simulink model "Batteryfault"  (R2021a)
settings: Solver=ode23t  StartTime=0.0  StopTime=50  RelTol=1e-3
libraries: ee_lib x40, fl_lib x12, nesl_utility x3
settings Model: Creator=perry  LastModifiedBy=perry

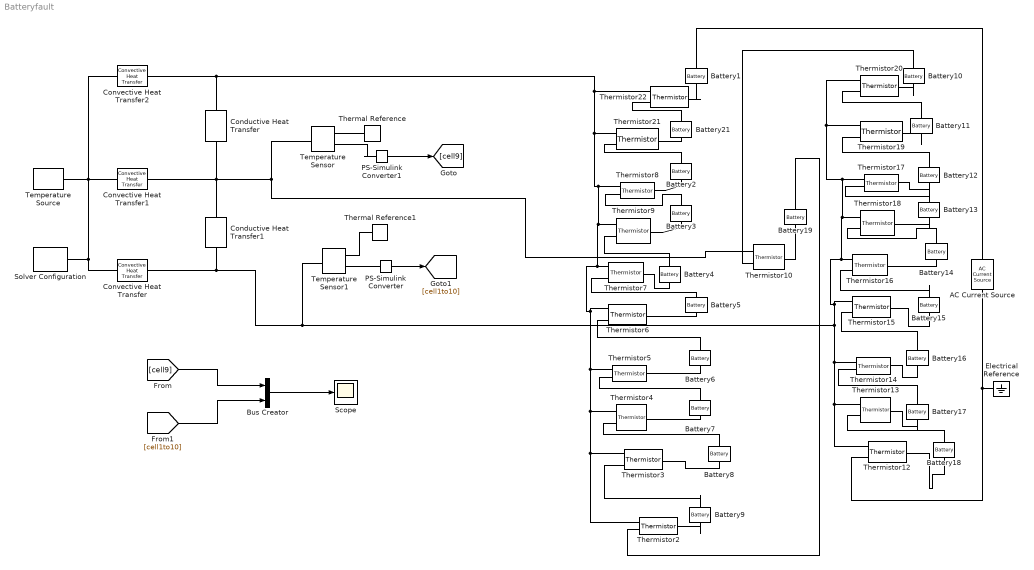
== system Batteryfault ==
  AC Current Source : fl_lib/Electrical/Electrical Sources/AC Current Source  amp=50 A  shift=0 deg  frequency=1/600 Hz  omega=0 rad/s
      settings: SourceProductBaseCode=SS  InternalSimscapePortConfiguration="{\"Bottom\":[],\"Left\":[{\"id\":\"p\",\"label\":\"\",\"type\":\"foundation.electrical.electrical\"}],\"Right\":[{\"id\":\"n\",\"label\":\"\",\"type\":\"foundation.electrical.electrical\"}],\"Top\":[]}"
  Battery{1..19,21} (20 alike) : ee_lib/Sources/Battery  Vnom=4 V  prm_dir=1  R1_dis=2 Ohm  R1_ch=2 Ohm  R1=0.001 Ohm  prm_AH=2  AH=5 hr*A  V1=3.6 V  AH1=4 hr*A  prm_R2=1  R2=2000 Ohm  prm_dyn=1  Rp1=0.005 Ohm  tau1=30 s  Rp2=0.005 Ohm  tau2=30 s  Rp3=0.005 Ohm  tau3=30 s  Rp4=0.005 Ohm  tau4=30 s  Rp5=0.005 Ohm  tau5=30 s  prm_fade=1  N_fade=100  AH_fade=45 hr*A  R1_fade=2.02 Ohm  R1_ch_fade=2.02 Ohm  V1_fade=10.35 V  prm_age=1  prm_age_OCV=1  OCV_age=0.9  SOC_age=60  Tmeas_age=298.15 K  delta_time_age_vec=[0] d  temperature_age_vec=[273] K  OCV_scaling_age=2.2134e6  OCV_offset_age=1.632e6  temp_exp_age=0.515833569 V  t_exp_age=0.75  i_specify=off  i_priority=None  i=0 A  i_nominal_specify=off  i_nominal_unit=A  i_nominal_value=1  v_specify=off  v_priority=None  v=0 V  v_nominal_specify=off  v_nominal_unit=V  v_nominal_value=1  charge_specify=off  charge_priority=High  charge=50 hr*A  charge_nominal_specify=off  charge_nominal_unit=hr*A  charge_nominal_value=1  num_cycles_specify=off  num_cycles_priority=High  num_cycles=0  num_cycles_nominal_specify=off  num_cycles_nominal_unit=1  num_cycles_nominal_value=1  thermal_mass=30000 J/K  Tmeas=298.15 K  Vnom_T2=12 V  R1_T2=2.2 Ohm  R1_T2_dis=2.2 Ohm  R1_T2_ch=2.2 Ohm  V1_T2=11.4 V  R2_T2=2200 Ohm  Rp1_T2=0.005 Ohm  tau1_T2=30 s  Rp2_T2=0.005 Ohm  tau2_T2=30 s  Rp3_T2=0.005 Ohm  tau3_T2=30 s  Rp4_T2=0.005 Ohm  tau4_T2=30 s  Rp5_T2=0.005 Ohm  tau5_T2=30 s  Tmeas2=273.15 K  temperature_specify=off  temperature_priority=High  temperature=298.15 K  temperature_nominal_specify=off  temperature_nominal_unit=K  temperature_nominal_value=1
      settings: SourceProductBaseCode=SN
  Bus Creator : BusCreator  Inputs=2
  Conductive Heat Transfer : fl_lib/Thermal/Thermal Elements/Conductive Heat Transfer  area=1e-4 m^2  thickness=0.1 m  th_cond=401 W/(m*K)  T_specify=off  T_priority=None  T=0 K  T_nominal_specify=off  T_nominal_unit=K  T_nominal_value=1  Q_specify=off  Q_priority=None  Q=0 W  Q_nominal_specify=off  Q_nominal_unit=W  Q_nominal_value=1
  Conductive Heat Transfer1 : fl_lib/Thermal/Thermal Elements/Conductive Heat Transfer  area=1e-4 m^2  thickness=0.1 m  th_cond=401 W/(m*K)  T_specify=off  T_priority=None  T=0 K  T_nominal_specify=off  T_nominal_unit=K  T_nominal_value=1  Q_specify=off  Q_priority=None  Q=0 W  Q_nominal_specify=off  Q_nominal_unit=W  Q_nominal_value=1
  Convective Heat Transfer : fl_lib/Thermal/Thermal Elements/Convective Heat Transfer  area=1e-4 m^2  heat_tr_coeff=20 W/(m^2 * K)  T_specify=off  T_priority=None  T=0 K  T_nominal_specify=off  T_nominal_unit=K  T_nominal_value=1  Q_specify=off  Q_priority=None  Q=0 W  Q_nominal_specify=off  Q_nominal_unit=W  Q_nominal_value=1
  Convective Heat Transfer1 : fl_lib/Thermal/Thermal Elements/Convective Heat Transfer  area=1e-4 m^2  heat_tr_coeff=20 W/(m^2 * K)  T_specify=off  T_priority=None  T=0 K  T_nominal_specify=off  T_nominal_unit=K  T_nominal_value=1  Q_specify=off  Q_priority=None  Q=0 W  Q_nominal_specify=off  Q_nominal_unit=W  Q_nominal_value=1
  Convective Heat Transfer2 : fl_lib/Thermal/Thermal Elements/Convective Heat Transfer  area=1e-4 m^2  heat_tr_coeff=20 W/(m^2 * K)  T_specify=off  T_priority=None  T=0 K  T_nominal_specify=off  T_nominal_unit=K  T_nominal_value=1  Q_specify=off  Q_priority=None  Q=0 W  Q_nominal_specify=off  Q_nominal_unit=W  Q_nominal_value=1
  Electrical Reference : fl_lib/Electrical/Electrical Elements/Electrical Reference
  PS-Simulink Converter : nesl_utility/PS-Simulink Converter  PhysicalDomain=network_engine_domain  SubClassName=ps_output  LeftPortType=input  RightPortType=output  PseudoPeriodic=off  Frequencies=[]  Unit=inherit  AffineConversion=off
      settings: SourceProductBaseCode=PW,SS
  PS-Simulink Converter1 : nesl_utility/PS-Simulink Converter  PhysicalDomain=network_engine_domain  SubClassName=ps_output  LeftPortType=input  RightPortType=output  PseudoPeriodic=off  Frequencies=[]  Unit=inherit  AffineConversion=off
      settings: SourceProductBaseCode=PW,SS
  Scope : Scope
  Solver Configuration : nesl_utility/Solver Configuration  PhysicalDomain=network_engine_domain  SubClassName=solver  LeftPortType=input  RightPortType=generic  Tones=[]  Harmonics=[]  SimulateNoise=off  Profile=off  UseLocalSampling=off  EnableSwitchedLinearOptims=on  FrequencyDomain=off  UseCCode=off  RelTol=0.001  AbsTol=1e-06  MinStep=1e-09  ToWorkspace=off  RevertToSquareIcSolve=off  NumHomotopyIterations=100  PhasorMode=off  PhasorModeNumHarmonics=1  DoDC=off  ResidualTolerance=1e-09  UseLocalSolver=off  LocalSolverChoice=NE_BACKWARD_EULER_ADVANCER  LocalSolverSampleTime=0.001  DoFixedCost=off  MaxNonlinIter=3  MaxModeIter=2  ComputeImpulses=off  ImpulseIterations=2  LinearAlgebra=Sparse  EquationFormulation=NE_TIME_EF  DelaysMemoryBudget=1024  AutomaticFiltering=on  FilteringTimeConstant=0.001  PartitionStorageMethod=AS_NEEDED  PartitionMemoryBudget=1024  PartitionMethod=ROBUST
      settings: SourceProductBaseCode=PW,SS
  Temperature Sensor : fl_lib/Thermal/Thermal Sensors/Temperature Sensor
  Temperature Sensor1 : fl_lib/Thermal/Thermal Sensors/Temperature Sensor
  Temperature Source : fl_lib/Thermal/Thermal Sources/Temperature Source  temperature=298 K
  Thermal Reference : fl_lib/Thermal/Thermal Elements/Thermal Reference
  Thermal Reference1 : fl_lib/Thermal/Thermal Elements/Thermal Reference
  Thermistor10 : ee_lib/Sensors & Transducers/Thermistor  R0=1000 Ohm  Bparam=3000 degC  T0=23 degC  tc=5.0 s  K_d=0.75e-3 W/K  T_specify=off  T_priority=High  T=298.15 K  T_nominal_specify=off  T_nominal_unit=K  T_nominal_value=1
      settings: SourceProductBaseCode=PS  InternalSimscapePortConfiguration="{\"Bottom\":[],\"Left\":[{\"id\":\"A\",\"label\":\"A\",\"type\":\"foundation.thermal.thermal\"},{\"id\":\"p\",\"label\":\"+\",\"type\":\"foundation.electrical.electrical\"}],\"Right\":[{\"id\":\"n\",\"label\":\"-\",\"type\":\"foundation.electrical.electrical\"}],\"Top\":[]}"
  Thermistor{2..9,12..22} (19 alike) : ee_lib/Sensors & Transducers/Thermistor  R0=1000 Ohm  Bparam=3000 degC  T0=25 degC  tc=5.0 s  K_d=0.75e-3 W/K  T_specify=off  T_priority=High  T=298.15 K  T_nominal_specify=off  T_nominal_unit=K  T_nominal_value=1
      settings: SourceProductBaseCode=PS  InternalSimscapePortConfiguration="{\"Bottom\":[],\"Left\":[{\"id\":\"A\",\"label\":\"A\",\"type\":\"foundation.thermal.thermal\"},{\"id\":\"p\",\"label\":\"+\",\"type\":\"foundation.electrical.electrical\"}],\"Right\":[{\"id\":\"n\",\"label\":\"-\",\"type\":\"foundation.electrical.electrical\"}],\"Top\":[]}"
  wires:
  PS-Simulink Converter1/1 -> [cell9]
  PS-Simulink Converter/1 -> [cell1to10]
  Bus Creator/1 -> Scope/1
  [cell9] -> Bus Creator/1
  [cell1to10] -> Bus Creator/2
  connections:
  Temperature Sensor1/RConn1 -- Thermal Reference1/LConn1
  Temperature Sensor1/RConn2 -- PS-Simulink Converter/LConn1
  Temperature Sensor/RConn1 -- Thermal Reference/LConn1
  PS-Simulink Converter1/LConn1 -- Temperature Sensor/RConn2
  Solver Configuration/RConn1 -- Convective Heat Transfer2/LConn1 -- Convective Heat Transfer1/LConn1 -- Temperature Source/LConn1 -- Convective Heat Transfer/LConn1
  Battery10/LConn1 -- Thermistor10/LConn2
  Battery10/RConn1 -- Thermistor20/RConn1
  Battery11/LConn1 -- Thermistor20/LConn2
  Battery11/RConn1 -- Thermistor19/RConn1
  Battery12/LConn1 -- Thermistor19/LConn2
  Thermistor17/RConn1 -- Battery12/RConn1
  Battery13/LConn1 -- Thermistor17/LConn2
  Battery13/RConn1 -- Thermistor18/RConn1
  Battery15/LConn1 -- Thermistor16/LConn2
  Battery15/RConn1 -- Thermistor15/RConn1
  Battery16/LConn1 -- Thermistor15/LConn2
  Battery16/RConn1 -- Thermistor14/RConn1
  Battery17/LConn1 -- Thermistor14/LConn2
  Battery17/RConn1 -- Thermistor13/RConn1
  Battery18/LConn1 -- Thermistor13/LConn2
  Battery18/RConn1 -- Thermistor12/RConn1
  AC Current Source/RConn1 -- Thermistor12/LConn2 -- Electrical Reference/LConn1
  Thermistor20/LConn1 -- Thermistor19/LConn1 -- Thermistor17/LConn1 -- Temperature Sensor1/LConn1 -- Convective Heat Transfer/RConn1 -- Conductive Heat Transfer1/RConn1 -- Thermistor12/LConn1 -- Thermistor13/LConn1 -- Thermistor14/LConn1 -- Thermistor15/LConn1 -- Thermistor16/LConn1 -- Thermistor18/LConn1
  Thermistor7/LConn1 -- Conductive Heat Transfer/LConn1 -- Convective Heat Transfer2/RConn1 -- Thermistor22/LConn1 -- Thermistor21/LConn1 -- Thermistor8/LConn1 -- Thermistor9/LConn1 -- Thermistor2/LConn1 -- Thermistor3/LConn1 -- Thermistor4/LConn1 -- Thermistor5/LConn1 -- Thermistor6/LConn1
  Thermistor22/RConn1 -- Battery1/RConn1
  Battery9/RConn1 -- Thermistor2/RConn1
  Thermistor21/RConn1 -- Battery21/RConn1
  Battery9/LConn1 -- Thermistor3/LConn2
  Battery21/LConn1 -- Thermistor22/LConn2
  Battery2/LConn1 -- Thermistor21/LConn2
  Thermistor8/RConn1 -- Battery2/RConn1
  Thermistor8/LConn2 -- Battery3/LConn1
  Thermistor9/RConn1 -- Battery3/RConn1
  Thermistor9/LConn2 -- Battery4/LConn1
  Thermistor7/RConn1 -- Battery4/RConn1
  Thermistor7/LConn2 -- Battery5/LConn1
  Thermistor6/RConn1 -- Battery5/RConn1
  Thermistor6/LConn2 -- Battery6/LConn1
  Thermistor5/RConn1 -- Battery6/RConn1
  Thermistor5/LConn2 -- Battery7/LConn1
  Thermistor4/RConn1 -- Battery7/RConn1
  Thermistor4/LConn2 -- Battery8/LConn1
  Thermistor3/RConn1 -- Battery8/RConn1
  Battery14/LConn1 -- Thermistor18/LConn2
  Thermistor16/RConn1 -- Battery14/RConn1
  Battery1/LConn1 -- AC Current Source/LConn1
  Convective Heat Transfer1/RConn1 -- Thermistor10/LConn1 -- Temperature Sensor/LConn1 -- Conductive Heat Transfer/RConn1 -- Conductive Heat Transfer1/LConn1
  Thermistor10/RConn1 -- Battery19/RConn1
  Battery19/LConn1 -- Thermistor2/LConn2
